simulink model "Test_UE_UAV"  (R2022b)
settings: Solver=VariableStepAuto  StartTime=0.0  StopTime=inf  RelTol=1e-3
undefined symbols (not defined in the file): Ts
libraries: simulink x12, visionsinks x2, sim3dcameralib x2, sim3dprobsensorlib x2, uavsim3dlib x2, simulink_extras x1, sim3dphyssensorlib x1, sim3dlib x1, sim3dgroundtruthsensorlib x1
settings Model: Creator=mluo  LastModifiedBy=mluo

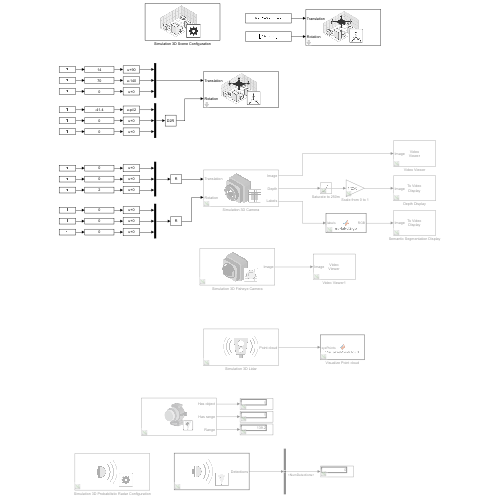
[thumbnail: Simulink's stored preview of the top-level diagram]
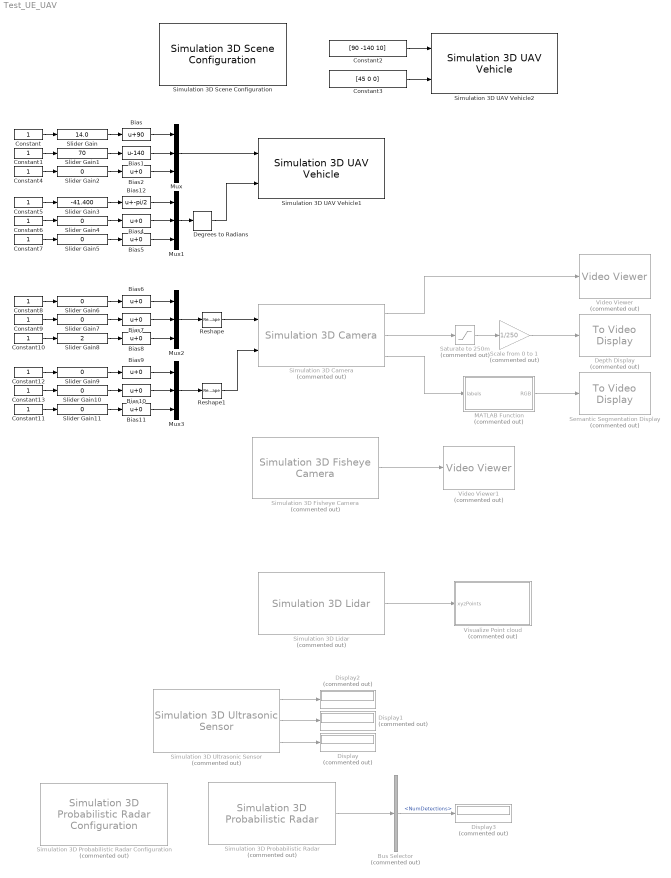
== system Test_UE_UAV ==
  Bias : Bias  Bias=90  SaturateOnIntegerOverflow=off
  Bias1 : Bias  Bias=-140  SaturateOnIntegerOverflow=off
  Bias{2,4..11} (9 alike) : Bias  SaturateOnIntegerOverflow=off
  Bias12 : Bias  Bias=-pi/2  SaturateOnIntegerOverflow=off
  Bus Selector : BusSelector  Commented=on  OutputSignals=NumDetections
  Constant{,1,4..13} (12 alike) : Constant
  Constant2 : Constant  Value=[90 -140 10]
  Constant3 : Constant  Value=[45 0 0]
  Degrees to Radians : simulink_extras/Transformations/Degrees to Radians
  Depth Display : visionsinks/To Video Display  Commented=on  windowSizeMode=Normal  openAtMdlStart=on  fullScreen=off  videoWindowX=497  videoWindowY=162  saveWindowSize=off  videoWindowWidth=1280  videoWindowHeight=720  inputColorFormat=RGB  inputType=Obsolete  imagePorts=One multidimensional signal  OutputDevice=On-screen video monitor  dataOrg=Column-major  isWindowOpen=off
  Display{,1..3} (4 alike) : Display  Commented=on
  MATLAB Function : MATLAB Function  Commented=on  TreatAsAtomicUnit=on
  Mux{,1..3} (4 alike) : Mux  Inputs=3
  Reshape : Reshape  OutputDimensionality=Customize  OutputDimensions=[1,3]
  Reshape1 : Reshape  OutputDimensionality=Customize  OutputDimensions=[1,3]
  Saturate to 250m : Saturate  Commented=on  UpperLimit=250  LowerLimit=0
  Scale from 0 to 1 : Gain  Commented=on  Gain=1/250
  Semantic Segmentation Display : visionsinks/To Video Display  Commented=on  windowSizeMode=Normal  openAtMdlStart=on  fullScreen=off  videoWindowX=538  videoWindowY=136  saveWindowSize=off  videoWindowWidth=1280  videoWindowHeight=720  inputColorFormat=RGB  inputType=Obsolete  imagePorts=One multidimensional signal  OutputDevice=On-screen video monitor  dataOrg=Column-major  isWindowOpen=off
  Simulation 3D Camera : sim3dcameralib/Simulation 3D Camera  Priority=1  Commented=on  sensorTag=Sim3dSensor1  sensorId=1  sensorName=Sim3dSensor1  vehTagList={'Scene Origin';'SimulinkVehicle1';'SimulinkVehicle2'}  vehTag=SimulinkVehicle2  mountLoc=Origin  offsetFlag=on  tmountOffset=[2, 0, 1]  extTmount=on  rmountOffset=[0, 0, 90]  extRmount=on  FocalLength=[1109, 1109]  OpticalCenter=[640, 360]  ImageSize=[720, 1280]  RadialDistortion=[0, 0]  TangentialDistortion=[0, 0]  SensorSkew=0  DepthOutportEnabled=on  SemanticOutportEnabled=on  TransformOutportEnabled=off  SampleTime=-1  mountPoint=[2 0 1]  mountOrientation=[0 0 -90]  aMode=4  ID=1
      settings: LibrarySourceBlock=uavsim3dlib/Simulation 3D Camera
  Simulation 3D Fisheye Camera : sim3dcameralib/Simulation 3D Fisheye Camera  Priority=1  Commented=on  sensorTag=Sim3dSensor5  sensorId=5  sensorName=Sim3dSensor5  vehTagList={'Scene Origin';'SimulinkVehicle1';'SimulinkVehicle2'}  vehTag=SimulinkVehicle2  mountLoc=Origin  offsetFlag=on  tmountOffset=[2, 3, 3]  extTmount=off  rmountOffset=[0, 0, 90]  extRmount=off  OpticalCenter=[640, 360]  ImageSize=[720, 1280]  RadialDistortion=[320, -0.0005, 0, 0]  StretchMatrix=[1, 0; 0, 1]  TransformOutportEnabled=off  SampleTime=-1  mountPoint=[2 -3 3]  mountOrientation=[0 0 -90]  aMode=4  ID=5
      settings: LibrarySourceBlock=uavsim3dlib/Simulation 3D Fisheye Camera
  Simulation 3D Lidar : sim3dphyssensorlib/Simulation 3D Lidar  Priority=1  Commented=on  sensorTag=Sim3dSensor2  sensorId=2  sensorName=Sim3dSensor2  vehTagList={'Scene Origin';'SimulinkVehicle1';'SimulinkVehicle2'}  vehTag=SimulinkVehicle2  mountLoc=Origin  offsetFlag=on  tmountOffset=[0, 20, 3]  rmountOffset=[0, 0, 90]  DetectionRange=300  RangeResolution=0.002  VerticalFOV=40  VerticalResolution=1.25  HorizontalFOV=360  HorizontalResolution=0.16  DistanceOutportEnabled=off  ReflectivityOutportEnabled=off  SemanticOutportEnabled=off  TransformOutportEnabled=off  SampleTime=-1  mountPoint=[0 -20 3]  mountOrientation=[0 0 -90]  aMode=4  ID=2
      settings: LibrarySourceBlock=uavsim3dlib/Simulation 3D Lidar
  Simulation 3D Probabilistic Radar : sim3dprobsensorlib/Simulation 3D Probabilistic Radar  Priority=1  Commented=on  sensorTag=Sim3dSensor4  sensorId=4  sensorName=Sim3dSensor4  vehTagList={'Scene Origin';'SimulinkVehicle1';'SimulinkVehicle2'}  vehTag=SimulinkVehicle2  mountLoc=Origin  offsetFlag=on  tmountOffset=[0, 0, 2]  rmountOffset=[0, 0, 0]  AzimuthResolution=1  ElevationResolution=1  RangeResolution=1  RangeRateResolution=0.5  AzimuthBiasFraction=0.1  ElevationBiasFraction=0.1  RangeBiasFraction=0.05  RangeRateBiasFraction=0.05  FieldOfView=[30, 5 ]  DetectionRange=[0.01, 150 ]  RangeRateLimits=[ -100, 100 ]  DetectionProbability=0.9  FalseAlarmRate=1e-6  ReferenceRange=150  ReferenceRCS=0  HasElevation=on  HasRangeRate=on  HasNoise=off  HasFalseAlarms=off  InitialSeedSource=Repeatable  InitialSeed=0  MaxNumDetections=10  DetectionCoordinates=Ego Cartesian  SpecifyOutputBusName=off  BusName=BusSimulation3DRadarTruthSensor  SampleTime=Ts  mountPoint=[0 0 2]  mountOrientation=[0 0 0]  aMode=3  ID=4
      settings: LibrarySourceBlock=drivingsim3d/Simulation 3D Probabilistic Radar
  Simulation 3D Probabilistic Radar Configuration : sim3dprobsensorlib/Simulation 3D Probabilistic Radar Configuration  Commented=on  RCSactorKeys=[10]  RCSactorProfiles={[10, 10;10, 10]}  RCSdefaultValue=-20  aMode=3
  Simulation 3D Scene Configuration : sim3dlib/Simulation 3D Scene Configuration  Priority=0  ProjectFormat=Unreal Editor  SceneDesc=US city block  ProjectName=C:\Program Files\MATLAB\R2022b\toolbox\shared\sim3d_projects\automotive_project\UE4\WindowsNoEditor\VehicleSimulation.exe  ScenePath=/Game/Maps/USCityBlock  UEProjPath=C:\OffRoad\StraddleCarrier\UnrealEngine\StraddleCarrier\StraddleCarrier.uproject  EnableOpenDRIVE=off  vehTagList={'Scene Origin';'SimulinkVehicle1';'SimulinkVehicle2'}  vehTag=SimulinkVehicle1  OpVisEn=off  Ts=Ts  EnableWindow=on  EnableRemoteAccess=off  EnableWeather=off  SunAltitude=60  SunAzimuth=200  clouds=20  wind=5  fog=0  rain=50  EnableGeospatial=off  OriginHeight=200  OriginLatitude=40.744652  OriginLongitude=-73.988864  MapStyle=Aerial  AdditionalAssetIDs=[]  UseAdvancedSunSky=off  SolarTime=11  TimeZone=-5  Day=21  Month=9  Year=2022  UseDaylightSavingTime=on  DSTStartDay=10  DSTStartMonth=3  DSTEndDay=3  DSTEndMonth=11  DSTSwitchHour=2  sensorTag=MainCamera1  sensorId=1  sensorName=MainCamera1  mountLoc=Origin  offsetFlag=off  tmountOffset=[0, 0, 0]  rmountOffset=[0, 0, 0]  HorizontalResolution=1280  VerticalResolution=720  HorizontalFOV=60  mountPoint=[0 0 0]  mountOrientation=[0 0 0]  aMode=4  ID=1  GeoTrigger=Inactive
      settings: LibrarySourceBlock=uavsim3dlib/Simulation 3D Scene Configuration
  Simulation 3D UAV Vehicle1 : uavsim3dlib/Simulation 3D UAV Vehicle  Priority=-1  Mesh=Custom  MeshPath=/MathWorksUAVContent/UAVs/Custom/Strad_UAV.Strad_UAV  Color=Black  ActorName=SimulinkVehicle2  InitialTranslation=[0 0 0]  InitialRotation=[0 0 0]  SampleTime=-1  ActorType=SimulinkVehicle  ID=2  aMode=4  ActorTag=SimulinkVehicle2
  Simulation 3D UAV Vehicle2 : uavsim3dlib/Simulation 3D UAV Vehicle  Priority=-1  Mesh=Custom  MeshPath=/MathWorksUAVContent/UAVs/Custom/Box.Box  Color=Black  ActorName=SimulinkVehicle1  InitialTranslation=[0 0 0]  InitialRotation=[0 0 0]  SampleTime=-1  ActorType=SimulinkVehicle  ID=1  aMode=4  ActorTag=SimulinkVehicle1
  Simulation 3D Ultrasonic Sensor : sim3dgroundtruthsensorlib/Simulation 3D Ultrasonic Sensor  Priority=1  Commented=on  sensorTag=Sim3dSensor3  sensorId=3  sensorName=Sim3dSensor3  vehTagList={'Scene Origin';'SimulinkVehicle1';'SimulinkVehicle2'}  vehTag=SimulinkVehicle2  mountLoc=Origin  offsetFlag=on  tmountOffset=[0, 0, 2]  rmountOffset=[0, 0, 90]  detectionRanges=[0.01 0.5 200]  HorizontalFoV=10  VerticalFoV=10  useBusOutput=off  SampleTime=-1  mountPoint=[0 0 2]  mountOrientation=[0 0 -90]  aMode=3  ID=3
      settings: LibrarySourceBlock=drivingsim3d/Simulation 3D Ultrasonic Sensor
  Slider Gain : simulink/Math Operations/Slider Gain  gain=14.0  low=-150  high=150
  Slider Gain1 : simulink/Math Operations/Slider Gain  gain=70  low=-150  high=150
  Slider Gain10 : simulink/Math Operations/Slider Gain  gain=0  low=-45  high=45
  Slider Gain11 : simulink/Math Operations/Slider Gain  gain=0  low=-45  high=45
  Slider Gain2 : simulink/Math Operations/Slider Gain  gain=0  low=-30  high=30
  Slider Gain3 : simulink/Math Operations/Slider Gain  gain=-41.400  low=-90  high=90
  Slider Gain4 : simulink/Math Operations/Slider Gain  gain=0  low=-30  high=30
  Slider Gain5 : simulink/Math Operations/Slider Gain  gain=0  low=-30  high=30
  Slider Gain6 : simulink/Math Operations/Slider Gain  gain=0  low=-5  high=5
  Slider Gain7 : simulink/Math Operations/Slider Gain  gain=0  low=-5  high=5
  Slider Gain8 : simulink/Math Operations/Slider Gain  gain=2  low=-5  high=5
  Slider Gain9 : simulink/Math Operations/Slider Gain  gain=0  low=-45  high=45
  Video Viewer : VideoViewer  Commented=on  FigPos=[1995 1113 1341 776]
  Video Viewer1 : VideoViewer  Commented=on  FigPos=[1995 1113 1341 776]
  Visualize Point cloud : MATLAB Function  Commented=on  StopFcn=|  TreatAsAtomicUnit=on
      | playerFigure = findall(groot,'type','figure','name','Point Cloud Player');
      | 
      | if ~isempty(playerFigure)
      |     playerFigure = playerFigure(end);
      |     if isvalid(playerFigure)
      |         close(playerFigure);
      |     end
      | end
  wires:
  Simulation 3D Camera/1 -> Video Viewer/1
  Simulation 3D Lidar/1 -> Visualize Point cloud/1(xyzPoints)
  Constant2/1 -> Simulation 3D UAV Vehicle2/1
  Constant3/1 -> Simulation 3D UAV Vehicle2/2
  Mux/1 -> Simulation 3D UAV Vehicle1/1
  Constant/1 -> Slider Gain/1
  Slider Gain/1 -> Bias/1
  Bias/1 -> Mux/1
  Constant1/1 -> Slider Gain1/1
  Slider Gain1/1 -> Bias1/1
  Bias1/1 -> Mux/2
  Constant4/1 -> Slider Gain2/1
  Slider Gain2/1 -> Bias2/1
  Bias2/1 -> Mux/3
  Slider Gain4/1 -> Bias4/1
  Constant6/1 -> Slider Gain4/1
  Bias4/1 -> Mux1/2
  Constant7/1 -> Slider Gain5/1
  Slider Gain5/1 -> Bias5/1
  Constant5/1 -> Slider Gain3/1
  Mux1/1 -> Degrees to Radians/1
  Bias5/1 -> Mux1/3
  Slider Gain3/1 -> Bias12/1
  Bias12/1 -> Mux1/1
  Degrees to Radians/1 -> Simulation 3D UAV Vehicle1/2
  Simulation 3D Ultrasonic Sensor/3 -> Display/1
  Simulation 3D Ultrasonic Sensor/2 -> Display1/1
  Simulation 3D Ultrasonic Sensor/1 -> Display2/1
  Simulation 3D Probabilistic Radar/1 -> Bus Selector/1
  Bus Selector/1 -> Display3/1  "<NumDetections>"
  Slider Gain7/1 -> Bias7/1
  Bias7/1 -> Mux2/2
  Constant8/1 -> Slider Gain6/1
  Constant10/1 -> Slider Gain8/1
  Slider Gain8/1 -> Bias8/1
  Bias8/1 -> Mux2/3
  Slider Gain6/1 -> Bias6/1
  Bias6/1 -> Mux2/1
  Constant9/1 -> Slider Gain7/1
  Mux2/1 -> Reshape/1
  Reshape/1 -> Simulation 3D Camera/1
  Constant13/1 -> Slider Gain10/1
  Constant11/1 -> Slider Gain11/1
  Bias9/1 -> Mux3/1
  Slider Gain10/1 -> Bias10/1
  Slider Gain9/1 -> Bias9/1
  Constant12/1 -> Slider Gain9/1
  Bias10/1 -> Mux3/2
  Slider Gain11/1 -> Bias11/1
  Bias11/1 -> Mux3/3
  Mux3/1 -> Reshape1/1
  Reshape1/1 -> Simulation 3D Camera/2
  Simulation 3D Camera/3 -> MATLAB Function/1(labels)
  Saturate to 250m/1 -> Scale from 0 to 1/1
  Simulation 3D Camera/2 -> Saturate to 250m/1
  Scale from 0 to 1/1 -> Depth Display/1
  MATLAB Function/1(RGB) -> Semantic Segmentation Display/1
  Simulation 3D Fisheye Camera/1 -> Video Viewer1/1

== matlab function Test_UE_UAV/Visualize Point cloud ==
  data: xyzPoints input
function VisualizePointCloud(xyzPoints)
%VisualizePointCloud Display point cloud

coder.extrinsic('isOpen', 'pcplayer')

persistent player;

if isempty(player)
    % Configure axes limits
    xlimits = [-90 90];
    ylimits = [-90 90];
    zlimits = [ -5 40];
    
    % Create a streaming Lidar viewer
    player = pcplayer(xlimits, ylimits, zlimits);
end

if ~isempty(player) && isOpen(player)
    view(player, xyzPoints);
end

== matlab function Test_UE_UAV/MATLAB Function ==
  data: labels input; RGB output
function RGB = uavlabel2rgb(labels)
% Convert semantic segmentation map captured during 3D simulation to RGB
% color image.

% Declare label2rgb function.
coder.extrinsic('label2rgb');

% Preallocate memory for RGB matrix.
RGB = coder.nullcopy(zeros(size(labels,1),size(labels,2),3,class(labels)));

% Define colormap using 3D simulation label IDs.
cmap = sim3dColormap;

% Convert labels to RGB color image.
RGB = label2rgb(labels, cmap);
